simulink model "DetailedHouse"  (R2025a)
settings: Solver=daessc  StartTime=0.0  StopTime=house.operational.datetime.simRunTimeSeconds  MaxStep=60  RelTol=1e-3
PreLoadFcn:
  | run("DetailedHouseParameters.mlx");
undefined symbols (not defined in the file or in its folder): house, value
libraries: fl_lib x36, nesl_utility x14, RoomVolume_lib x12, ExternalWall_lib x5, SolarRadiationAtLocation_lib x1, TemperatureSource_lib x1
CloseFcn:
  | clear house
settings Model: Creator=vikrants  LastModifiedBy=asakhare
settings DataIOCC: ReturnWorkspaceOutputsName=DetailedHouseSimResults

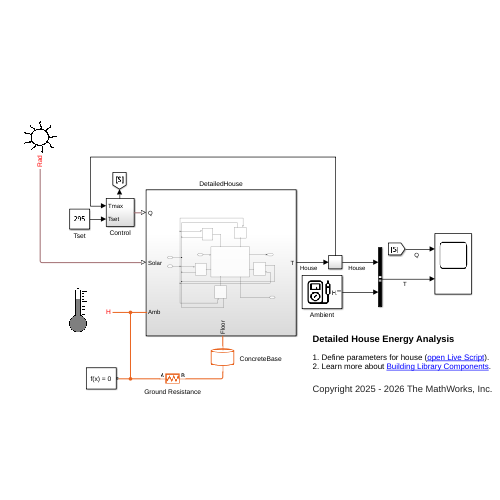
[thumbnail: Simulink's stored preview of the top-level diagram]
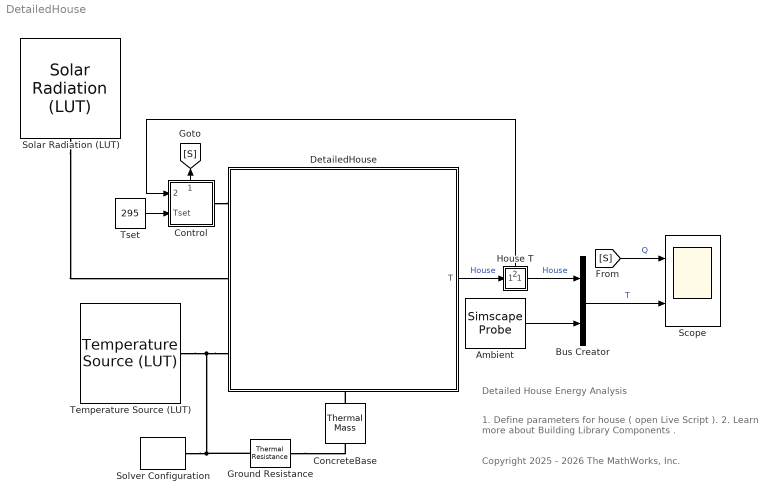
== system DetailedHouse ==
  note: 1. Define parameters for house ( open Live Script ).
      | 2. Learn more about Building Library Components .
  note: Copyright 2025 - 2026 The MathWorks, Inc.
  note: Detailed House Energy Analysis
  Ambient : SimscapeProbe  BoundBlock=326  Variables={H.T}
  Bus Creator : BusCreator  Inputs=2
  ConcreteBase : fl_lib/Thermal/Thermal Elements/Thermal Mass  mass_type=foundation.enum.constant_variable.constant  mass=1000 kg  sp_heat=447 J/(K*kg)  mass_min=1e-6 kg  num_ports=foundation.enum.numPorts2.two  m_specify=off  m_priority=High  m=1 kg  m_nominal_specify=off  m_nominal_value=1  m_nominal_unit=kg  T_specify=on  T_priority=High  T="value(house.heatTransfer.initialT,\"K\") K"  T_nominal_specify=off  T_nominal_value=1  T_nominal_unit=K  Q_specify=off  Q_priority=None  Q=0 W  Q_nominal_specify=off  Q_nominal_value=1  Q_nominal_unit=W
      settings: InternalSimscapePortConfiguration="{\"Bottom\":[],\"Left\":[{\"id\":\"M\",\"label\":\"\",\"type\":\"foundation.thermal.thermal\"}],\"Right\":[{\"id\":\"N\",\"label\":\"\",\"type\":\"foundation.thermal.thermal\"}],\"Top\":[]}"
  Control : Subsystem
      settings: PortSchema="{\"entries\":[{\"content\":{\"sides\":[{\"content\":{\"connectorIds\":[\"LConn1\"]},\"type\":\"ConnectorPlacement.EquallySpacedRectSide\",\"uuid\":\"bf0d3f6c-4199-48ed-9d1b-942d678a196d\"},{\"content\":{\"connectorIds\":[\"In1\",\"In2\"],\"side\":\"RIGHT\"},\"type\":\"ConnectorPlacement.EquallySpacedRectSide\",\"uuid\":\"048b5b2b-ccfc-4083-80b1-51c1896923e2\"},{\"content\":{\"side\":\"TOP\"},\"type\":\"ConnectorPlacement.EquallySpacedRectSide\",\"uuid\":\"550f74ea-2758-4466-8134-2f10276d8ab6\"},{\"content\":{\"connectorIds\":[\"Out1\"],\"side\":\"BOTTOM\"},\"type\":\"ConnectorPlacement.EquallySpacedRectSide\",\"uuid\":\"b8e21315-4710-4fb3-a2ab-c08e79356caa\"}]},\"type\":\"ConnectorPlacement.EquallySpacedConnector\",\"uuid\":\"91aadc23-894a-4dd0-ab72-650090e5f490\"}],\"packageUris\":[\"http://schema.mathworks.com/mf0/Connector/R2020b\"],\"version\":\"1.0\"}"
  DetailedHouse : Subsystem
      settings: PortSchema="{\"entries\":[{\"content\":{\"sides\":[{\"content\":{\"connectorIds\":[\"LConn1\",\"LConn2\",\"LConn3\"]},\"type\":\"ConnectorPlacement.EquallySpacedRectSide\",\"uuid\":\"299cb99e-37c4-4363-a148-c4e2a80bfd54\"},{\"content\":{\"connectorIds\":[\"Out1\"],\"side\":\"RIGHT\"},\"type\":\"ConnectorPlacement.EquallySpacedRectSide\",\"uuid\":\"2fcdd946-1002-4526-8c08-99e8dc6f4c47\"},{\"content\":{\"side\":\"TOP\"},\"type\":\"ConnectorPlacement.EquallySpacedRectSide\",\"uuid\":\"2d615648-e660-4e83-8c42-1b0b4f8091a8\"},{\"content\":{\"connectorIds\":[\"RConn1\"],\"side\":\"BOTTOM\"},\"type\":\"ConnectorPlacement.EquallySpacedRectSide\",\"uuid\":\"84e055a1-92e7-4959-a6d0-9bd398da1db3\"}]},\"type\":\"ConnectorPlacement.EquallySpacedConnector\",\"uuid\":\"3ed9db10-44da-4b23-b671-8dba5af5dcc9\"}],\"packageUris\":[\"http://schema.mathworks.com/mf0/Connector/R2020b\"],\"version\":\"1.0\"}"
  Ground Resistance : fl_lib/Thermal/Thermal Elements/Thermal Resistance  resistance=100 K/W  T_specify=off  T_priority=None  T=0 K  T_nominal_specify=off  T_nominal_value=1  T_nominal_unit=K  Q_specify=off  Q_priority=None  Q=0 W  Q_nominal_specify=off  Q_nominal_value=1  Q_nominal_unit=W
  House T : Subsystem
      settings: PortSchema="{\"entries\":[{\"content\":{\"sides\":[{\"content\":{\"connectorIds\":[\"In1\"]},\"type\":\"ConnectorPlacement.EquallySpacedRectSide\",\"uuid\":\"77a9471e-f475-4272-a324-d9a4c745a553\"},{\"content\":{\"connectorIds\":[\"Out1\"],\"side\":\"RIGHT\"},\"type\":\"ConnectorPlacement.EquallySpacedRectSide\",\"uuid\":\"144991d0-730c-43fd-a2ae-35995e9102ff\"},{\"content\":{\"connectorIds\":[\"Out2\"],\"side\":\"TOP\"},\"type\":\"ConnectorPlacement.EquallySpacedRectSide\",\"uuid\":\"5bc365e2-0ae2-46a9-8284-20be403f9731\"}]},\"type\":\"ConnectorPlacement.EquallySpacedConnector\",\"uuid\":\"845681d4-4f1f-48ee-9a7c-95a2152e9ae6\"}],\"packageUris\":[\"http://schema.mathworks.com/mf0/Connector/R2020b\"],\"version\":\"1.0\"}"
  Scope : Scope  NumInputPorts=2
      settings: ActiveDisplayYMinimum=-520.83333333333337  ActiveDisplayYMaximum=520.83333333333337  YLabel=Q  DataLoggingVariableName=DetailedHouseScopeData
  Solar Radiation (LUT) : SolarRadiationAtLocation_lib/Solar Radiation (LUT)  latitude=house.operational.location.latitude  longitude=house.operational.location.longitude  localTime=house.operational.location.localTime  dayLightS=house.operational.location.daylight  startYear=house.operational.datetime.year  startMonth=house.operational.datetime.month  startDay=house.operational.datetime.day  startHr=house.operational.datetime.hour  numHrsData=house.operational.datetime.numOfHourData  cloudData=cloudCoverLibOption.none  cloudCoverVal=ones(1,ceil(721/24))  interp_method=simscape.enum.interpolation.linear  extrap_method=simscape.enum.extrapolation.nearest
      settings: SourceProductName=Simscape Building Energy Management System Library  InternalSimscapePortConfiguration="{\"Bottom\":[],\"Left\":[],\"Right\":[{\"id\":\"S\",\"label\":\"Rad\",\"type\":\"output\"}],\"Top\":[]}"
  Solver Configuration : nesl_utility/Solver Configuration  PhysicalDomain=network_engine_domain  SubClassName=solver  LeftPortType=input  RightPortType=generic  Tones=[]  Harmonics=[]  SimulateNoise=off  Profile=off  UseLocalSampling=off  EnableSwitchedLinearOptims=on  FrequencyDomain=off  UseCCode=off  RelTol=0.001  AbsTol=0.001  MinStep=1e-09  ToWorkspace=off  RevertToSquareIcSolve=off  NumHomotopyIterations=100  PhasorMode=off  PhasorModeNumHarmonics=1  ConsistencySolver=NEWTON_XTOL_AFTER_FTOL  IndexReductionMethod=DerivativeReplacement  DoDC=off  ResidualTolerance=1e-09  ConsistencyTolSource=GLOBAL  ConsistencyAbsTol=0.001  ConsistencyRelTol=0.001  ConsistencyTolFactor=0.001  UseLocalSolver=off  LocalSolverChoice=NE_BACKWARD_EULER_ADVANCER  ResolveIndetEquations=on  FunctionEvalNumThread=1  LocalSolverSampleTime=0.001  DoFixedCost=off  MaxNonlinIter=3  MaxModeIter=2  ComputeImpulses=off  ImpulseIterations=2  LinearAlgebra=auto  LinearAlgebraNumThread=0  EquationFormulation=NE_TIME_EF  DelaysMemoryBudget=1024  AutomaticFiltering=on  FilteringTimeConstant=0.001  PartitionStorageMethod=AS_NEEDED  PartitionMemoryBudget=1024  PartitionMethod=ROBUST  MultibodyUseLocalSolver=off  MultibodyLocalSolverChoice=ODE1  MultibodyLocalSolverSampleTime=0.001
  Temperature Source (LUT) : TemperatureSource_lib/Temperature Source (LUT)  latitude=house.operational.location.latitude  longitude=house.operational.location.longitude  localTime=house.operational.location.localTime  dayLightS=house.operational.location.daylight  startYear=house.operational.datetime.year  startMonth=house.operational.datetime.month  startDay=house.operational.datetime.day  startHr=house.operational.datetime.hour  numDaysData=house.operational.datetime.numOfDaysData  interp_method=simscape.enum.interpolation.linear  extrap_method=simscape.enum.extrapolation.error  avgDayTvec="value(house.heatTransfer.avgDayTvec,\"K\") K"  pcDayTvar=house.heatTransfer.avgDayTvar  avgNightTvec="value(house.heatTransfer.avgNightTvec,\"K\") K"  pcNightTvar=house.heatTransfer.avgNightTvar
      settings: InternalSimscapePortConfiguration="{\"Bottom\":[],\"Left\":[],\"Right\":[{\"id\":\"H\",\"label\":\"H\",\"type\":\"foundation.thermal.thermal\"}],\"Top\":[]}"
  Tset : Constant  Value=295
  wires:
  DetailedHouse/1(T) -> House T/1(" ")  "House"
  House T/2("    ") -> Control/2(Tmax)
  Tset/1 -> Control/1(Tset)
  Control/1(" ") -> [S]
  Bus Creator/1 -> Scope/2  "T"
  House T/1("  ") -> Bus Creator/1  "House"
  [S] -> Scope/1  "Q"
  Ambient/1 -> Bus Creator/2
  connections:
  Solar Radiation (LUT)/RConn1 -- DetailedHouse/LConn2
  DetailedHouse/LConn3 -- Solver Configuration/RConn1 -- Ground Resistance/LConn1 -- Temperature Source (LUT)/RConn1
  ConcreteBase/LConn1 -- DetailedHouse/RConn1
  Ground Resistance/RConn1 -- ConcreteBase/RConn1
  Control/LConn1 -- DetailedHouse/LConn1

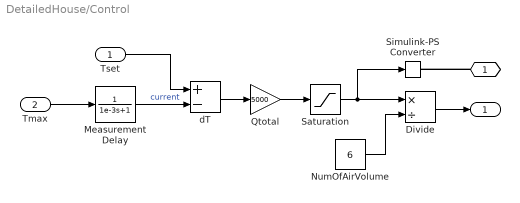
== system DetailedHouse/Control ==
  Tset : Inport
  Tmax : Inport  Port=2
  Divide : Product  Inputs=*/
  Measurement Delay : TransferFcn  Denominator=[1e-3 1]
  NumOfAirVolume : Constant  Value=6
  Qtotal : Gain  Gain=5000
  Saturation : Saturate  UpperLimit=2500  LowerLimit=-2500
  Simulink-PS Converter : nesl_utility/Simulink-PS Converter  PhysicalDomain=network_engine_domain  SubClassName=ps_input  LeftPortType=input  RightPortType=output  PseudoPeriodic=off  Frequencies=[]  NoiseDistribution=none  NoiseParameters=[]  Unit=J/s  AffineConversion=off  FilteringAndDerivatives=provide  SimscapeFilterOrder=1  InputFilterTimeConstant=0.001  UdotUserProvided=0
  dT : Sum  Inputs=+-
  "  " : PMIOPort  Side=Left
  " " : Outport
  wires:
  Tset/1 -> dT/1
  dT/1 -> Qtotal/1
  Qtotal/1 -> Saturation/1
  Saturation/1 -> Divide/1, Simulink-PS Converter/1
  Tmax/1 -> Measurement Delay/1
  Measurement Delay/1 -> dT/2  "current"
  Divide/1 -> " "/1
  NumOfAirVolume/1 -> Divide/2
  connections:
  "  "/RConn1 -- Simulink-PS Converter/RConn1

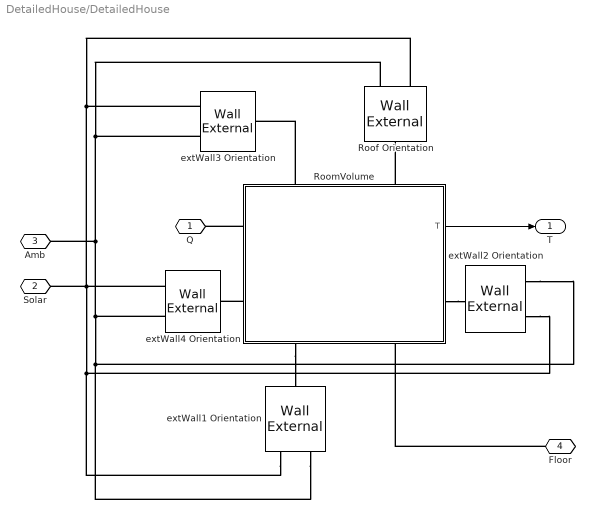
== system DetailedHouse/DetailedHouse ==
  Roof Orientation : ExternalWall_lib/Wall External  extWallModel=wallExternalModelOption.wallSolar  wallLength="value(house.lengthX,\"m\"); m"  wallHeight="value(house.lengthY,\"m\"); m"  wallThickness="house.wall.properties(\"Thickness [m]\",\"Roof\").Variables m"  wallMaterialDen="house.wall.properties(\"Density [kg/m^3]\",\"Roof\").Variables kg/m^3"  wallMaterialCp="house.wall.properties(\"Heat Capacity [J/kg-K]\",\"Roof\").Variables J/(K*kg)"  wallAbsorptivity="house.wall.properties(\"Absorptivity [-]\",\"Roof\").Variables"  wallThermalK="house.wall.properties(\"Thermal Conductivity [W/K-m]\",\"Roof\").Variables W/(K*m)"  winLength=1 m  winHeight=0.5 m  winThickness=0.007 m  winMaterialDen=2500 kg/m^3  winMaterialCp=787 J/(K*kg)  winAbsorptivity=0.35  winThermalK=1 W/(K*m)  winTransmissivity=0.45  ventLength=0.1 m  ventHeight=0.1 m  extToWallHTC="value(house.heatTransfer.externalHTC,\"W/(K*m^2)\") W/(K*m^2)"  intToRoomHTC="value(house.heatTransfer.htc,\"W/(K*m^2)\") W/(K*m^2)"  iniT="value(house.heatTransfer.initialT,\"K\") K"  latitude=house.operational.location.latitude  longitude=house.operational.location.longitude  localTime=house.operational.location.localTime  dayLightS=house.operational.location.daylight  surfAngle=0 deg  surfUnitV=[0, -1]  startYear=house.operational.datetime.year  startMonth=house.operational.datetime.month  startDay=house.operational.datetime.day  startHr=house.operational.datetime.hour  numHrsData=house.operational.datetime.numOfHourData  interp_method=simscape.enum.interpolation.linear  extrap_method=simscape.enum.extrapolation.error
      settings: InternalSimscapePortConfiguration="{\"Bottom\":[],\"Left\":[{\"id\":\"R\",\"label\":\"Rad\",\"type\":\"input\"},{\"id\":\"A\",\"label\":\"A\",\"type\":\"foundation.thermal.thermal\"}],\"Right\":[{\"id\":\"B\",\"label\":\"B\",\"type\":\"foundation.thermal.thermal\"}],\"Top\":[]}"
  RoomVolume : Subsystem
      settings: PortSchema="{\"entries\":[{\"content\":{\"sides\":[{\"content\":{\"connectorIds\":[\"LConn1\",\"LConn2\"]},\"type\":\"ConnectorPlacement.EquallySpacedRectSide\",\"uuid\":\"bb55eb80-d4a7-43ce-a7a0-972e6a4ef911\"},{\"content\":{\"connectorIds\":[\"Out1\",\"RConn1\"],\"side\":\"RIGHT\"},\"type\":\"ConnectorPlacement.EquallySpacedRectSide\",\"uuid\":\"29951cfd-9715-464b-88ca-0c0ac5d49cc2\"},{\"content\":{\"connectorIds\":[\"LConn3\",\"LConn4\"],\"side\":\"TOP\"},\"type\":\"ConnectorPlacement.EquallySpacedRectSide\",\"uuid\":\"a06c10be-0f38-432f-83ff-ea95edd1594a\"},{\"content\":{\"connectorIds\":[\"RConn2\",\"RConn3\"],\"side\":\"BOTTOM\"},\"type\":\"ConnectorPlacement.EquallySpacedRectSide\",\"uuid\":\"c57a9caa-6d36-48ec-a075-3784b3a7d3f9\"}]},\"type\":\"ConnectorPlacement.EquallySpacedConnector\",\"uuid\":\"940ec8b0-d9b9-4e36-b0c1-d94fb2f52aba\"}],\"packageUris\":[\"http://schema.mathworks.com/mf0/Connector/R2020b\"],\"version\":\"1.0\"}"
  extWall1 Orientation : ExternalWall_lib/Wall External  extWallModel=wallExternalModelOption.wallSolarWinVent  wallLength="value(house.lengthX,\"m\") m"  wallHeight="value(house.lengthZ,\"m\") m"  wallThickness="house.wall.properties(\"Thickness [m]\",\"ExternalWall\").Variables m"  wallMaterialDen="house.wall.properties(\"Density [kg/m^3]\",\"ExternalWall\").Variables kg/m^3"  wallMaterialCp="house.wall.properties(\"Heat Capacity [J/kg-K]\",\"ExternalWall\").Variables J/(K*kg)"  wallAbsorptivity="house.wall.properties(\"Absorptivity [-]\",\"ExternalWall\").Variables"  wallThermalK="house.wall.properties(\"Thermal Conductivity [W/K-m]\",\"ExternalWall\").Variables W/(K*m)"  winLength="sqrt(house.wall.opening.window)*value(house.lengthX,\"m\") m"  winHeight="sqrt(house.wall.opening.window)*value(house.lengthZ,\"m\") m"  winThickness="house.wall.properties(\"Thickness [m]\",\"Window\").Variables m"  winMaterialDen="house.wall.properties(\"Density [kg/m^3]\",\"Window\").Variables kg/m^3"  winMaterialCp="house.wall.properties(\"Heat Capacity [J/kg-K]\",\"Window\").Variables J/(K*kg)"  winAbsorptivity="house.wall.properties(\"Absorptivity [-]\",\"Window\").Variables"  winThermalK="house.wall.properties(\"Thermal Conductivity [W/K-m]\",\"Window\").Variables W/(K*m)"  winTransmissivity="house.wall.properties(\"Transmissivity [-]\",\"Window\").Variables"  ventLength="sqrt(house.wall.opening.vent)*value(house.lengthX,\"m\") m"  ventHeight="sqrt(house.wall.opening.vent)*value(house.lengthZ,\"m\") m"  extToWallHTC="value(house.heatTransfer.externalHTC,\"W/(K*m^2)\") W/(K*m^2)"  intToRoomHTC="value(house.heatTransfer.htc,\"W/(K*m^2)\") W/(K*m^2)"  iniT="value(house.heatTransfer.initialT,\"K\") K"  latitude=house.operational.location.latitude  longitude=house.operational.location.longitude  localTime=house.operational.location.localTime  dayLightS=house.operational.location.daylight  surfAngle=90 deg  surfUnitV=[0, -1]  startYear=house.operational.datetime.year  startMonth=house.operational.datetime.month  startDay=house.operational.datetime.day  startHr=house.operational.datetime.hour  numHrsData=house.operational.datetime.numOfHourData  interp_method=simscape.enum.interpolation.linear  extrap_method=simscape.enum.extrapolation.error
      settings: InternalSimscapePortConfiguration="{\"Bottom\":[],\"Left\":[{\"id\":\"R\",\"label\":\"Rad\",\"type\":\"input\"},{\"id\":\"A\",\"label\":\"A\",\"type\":\"foundation.thermal.thermal\"}],\"Right\":[{\"id\":\"B\",\"label\":\"B\",\"type\":\"foundation.thermal.thermal\"}],\"Top\":[]}"
  extWall2 Orientation : ExternalWall_lib/Wall External  extWallModel=wallExternalModelOption.wallSolarVent  wallLength="value(house.lengthY,\"m\"); m"  wallHeight="value(house.lengthZ,\"m\"); m"  wallThickness="house.wall.properties(\"Thickness [m]\",\"ExternalWall\").Variables m"  wallMaterialDen="house.wall.properties(\"Density [kg/m^3]\",\"ExternalWall\").Variables kg/m^3"  wallMaterialCp="house.wall.properties(\"Heat Capacity [J/kg-K]\",\"ExternalWall\").Variables J/(K*kg)"  wallAbsorptivity="house.wall.properties(\"Absorptivity [-]\",\"ExternalWall\").Variables"  wallThermalK="house.wall.properties(\"Thermal Conductivity [W/K-m]\",\"ExternalWall\").Variables W/(K*m)"  winLength=1 m  winHeight=0.5 m  winThickness=0.007 m  winMaterialDen=2500 kg/m^3  winMaterialCp=787 J/(K*kg)  winAbsorptivity=0.35  winThermalK=1 W/(K*m)  winTransmissivity=0.45  ventLength="sqrt(house.wall.opening.vent)*value(house.lengthY,\"m\") m"  ventHeight="sqrt(house.wall.opening.vent)*value(house.lengthZ,\"m\") m"  extToWallHTC="value(house.heatTransfer.externalHTC,\"W/(K*m^2)\") W/(K*m^2)"  intToRoomHTC="value(house.heatTransfer.htc,\"W/(K*m^2)\") W/(K*m^2)"  iniT="value(house.heatTransfer.initialT,\"K\") K"  latitude=house.operational.location.latitude  longitude=house.operational.location.longitude  localTime=house.operational.location.localTime  dayLightS=house.operational.location.daylight  surfAngle=90 deg  surfUnitV=[1,0]  startYear=house.operational.datetime.year  startMonth=house.operational.datetime.month  startDay=house.operational.datetime.day  startHr=house.operational.datetime.hour  numHrsData=house.operational.datetime.numOfHourData  interp_method=simscape.enum.interpolation.linear  extrap_method=simscape.enum.extrapolation.error
      settings: InternalSimscapePortConfiguration="{\"Bottom\":[],\"Left\":[{\"id\":\"R\",\"label\":\"Rad\",\"type\":\"input\"},{\"id\":\"A\",\"label\":\"A\",\"type\":\"foundation.thermal.thermal\"}],\"Right\":[{\"id\":\"B\",\"label\":\"B\",\"type\":\"foundation.thermal.thermal\"}],\"Top\":[]}"
  extWall3 Orientation : ExternalWall_lib/Wall External  extWallModel=wallExternalModelOption.wallSolar  wallLength="value(house.lengthX,\"m\"); m"  wallHeight="value(house.lengthZ,\"m\"); m"  wallThickness="house.wall.properties(\"Thickness [m]\",\"ExternalWall\").Variables m"  wallMaterialDen="house.wall.properties(\"Density [kg/m^3]\",\"ExternalWall\").Variables kg/m^3"  wallMaterialCp="house.wall.properties(\"Heat Capacity [J/kg-K]\",\"ExternalWall\").Variables J/(K*kg)"  wallAbsorptivity="house.wall.properties(\"Absorptivity [-]\",\"ExternalWall\").Variables"  wallThermalK="house.wall.properties(\"Thermal Conductivity [W/K-m]\",\"ExternalWall\").Variables W/(K*m)"  winLength=1 m  winHeight=0.5 m  winThickness=0.007 m  winMaterialDen=2500 kg/m^3  winMaterialCp=787 J/(K*kg)  winAbsorptivity=0.35  winThermalK=1 W/(K*m)  winTransmissivity=0.45  ventLength=0.1 m  ventHeight=0.1 m  extToWallHTC="value(house.heatTransfer.externalHTC,\"W/(K*m^2)\") W/(K*m^2)"  intToRoomHTC="value(house.heatTransfer.htc,\"W/(K*m^2)\") W/(K*m^2)"  iniT="value(house.heatTransfer.initialT,\"K\") K"  latitude=house.operational.location.latitude  longitude=house.operational.location.longitude  localTime=house.operational.location.localTime  dayLightS=house.operational.location.daylight  surfAngle=90 deg  surfUnitV=[0, 1]  startYear=house.operational.datetime.year  startMonth=house.operational.datetime.month  startDay=house.operational.datetime.day  startHr=house.operational.datetime.hour  numHrsData=house.operational.datetime.numOfHourData  interp_method=simscape.enum.interpolation.linear  extrap_method=simscape.enum.extrapolation.error
      settings: InternalSimscapePortConfiguration="{\"Bottom\":[],\"Left\":[{\"id\":\"R\",\"label\":\"Rad\",\"type\":\"input\"},{\"id\":\"A\",\"label\":\"A\",\"type\":\"foundation.thermal.thermal\"}],\"Right\":[{\"id\":\"B\",\"label\":\"B\",\"type\":\"foundation.thermal.thermal\"}],\"Top\":[]}"
  extWall4 Orientation : ExternalWall_lib/Wall External  extWallModel=wallExternalModelOption.wallSolarWin  wallLength="value(house.lengthY,\"m\"); m"  wallHeight="value(house.lengthZ,\"m\"); m"  wallThickness="house.wall.properties(\"Thickness [m]\",\"ExternalWall\").Variables m"  wallMaterialDen="house.wall.properties(\"Density [kg/m^3]\",\"ExternalWall\").Variables kg/m^3"  wallMaterialCp="house.wall.properties(\"Heat Capacity [J/kg-K]\",\"ExternalWall\").Variables J/(K*kg)"  wallAbsorptivity="house.wall.properties(\"Absorptivity [-]\",\"ExternalWall\").Variables"  wallThermalK="house.wall.properties(\"Thermal Conductivity [W/K-m]\",\"ExternalWall\").Variables W/(K*m)"  winLength="sqrt(house.wall.opening.window)*value(house.lengthY,\"m\") m"  winHeight="sqrt(house.wall.opening.window)*value(house.lengthZ,\"m\") m"  winThickness="house.wall.properties(\"Thickness [m]\",\"Window\").Variables m"  winMaterialDen="house.wall.properties(\"Density [kg/m^3]\",\"Window\").Variables kg/m^3"  winMaterialCp="house.wall.properties(\"Heat Capacity [J/kg-K]\",\"Window\").Variables J/(K*kg)"  winAbsorptivity="house.wall.properties(\"Absorptivity [-]\",\"Window\").Variables"  winThermalK="house.wall.properties(\"Thermal Conductivity [W/K-m]\",\"Window\").Variables W/(K*m)"  winTransmissivity="house.wall.properties(\"Transmissivity [-]\",\"Window\").Variables"  ventLength=0.1 m  ventHeight=0.1 m  extToWallHTC="value(house.heatTransfer.externalHTC,\"W/(K*m^2)\") W/(K*m^2)"  intToRoomHTC="value(house.heatTransfer.htc,\"W/(K*m^2)\") W/(K*m^2)"  iniT="value(house.heatTransfer.initialT,\"K\") K"  latitude=house.operational.location.latitude  longitude=house.operational.location.longitude  localTime=house.operational.location.localTime  dayLightS=house.operational.location.daylight  surfAngle=90 deg  surfUnitV=[-1,0]  startYear=house.operational.datetime.year  startMonth=house.operational.datetime.month  startDay=house.operational.datetime.day  startHr=house.operational.datetime.hour  numHrsData=house.operational.datetime.numOfHourData  interp_method=simscape.enum.interpolation.linear  extrap_method=simscape.enum.extrapolation.error
      settings: InternalSimscapePortConfiguration="{\"Bottom\":[],\"Left\":[{\"id\":\"R\",\"label\":\"Rad\",\"type\":\"input\"},{\"id\":\"A\",\"label\":\"A\",\"type\":\"foundation.thermal.thermal\"}],\"Right\":[{\"id\":\"B\",\"label\":\"B\",\"type\":\"foundation.thermal.thermal\"}],\"Top\":[]}"
  Q : PMIOPort  Side=Left
  Solar : PMIOPort  Port=2  Side=Left
  Amb : PMIOPort  Port=3  Side=Left
  Floor : PMIOPort  Port=4  Side=Right
  T : Outport
  wires:
  RoomVolume/1(T) -> T/1
  connections:
  RoomVolume/LConn1 -- Q/RConn1
  Roof Orientation/LConn2 -- extWall2 Orientation/LConn2 -- extWall1 Orientation/LConn2 -- extWall4 Orientation/LConn2 -- Amb/RConn1 -- extWall3 Orientation/LConn2
  RoomVolume/LConn4 -- Roof Orientation/RConn1
  Solar/RConn1 -- extWall3 Orientation/LConn1 -- Roof Orientation/LConn1 -- extWall4 Orientation/LConn1 -- extWall2 Orientation/LConn1 -- extWall1 Orientation/LConn1
  RoomVolume/RConn2 -- extWall1 Orientation/RConn1
  RoomVolume/RConn1 -- extWall2 Orientation/RConn1
  RoomVolume/LConn3 -- extWall3 Orientation/RConn1
  RoomVolume/LConn2 -- extWall4 Orientation/RConn1
  Floor/RConn1 -- RoomVolume/RConn3

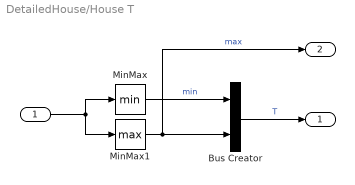
== system DetailedHouse/House T ==
  " " : Inport
  Bus Creator : BusCreator  Inputs=2
  MinMax : MinMax
  MinMax1 : MinMax  Function=max
  "  " : Outport
  "    " : Outport  Port=2
  wires:
  MinMax1/1 -> "    "/1, Bus Creator/2  "max"
  MinMax/1 -> Bus Creator/1  "min"
  " "/1 -> MinMax/1, MinMax1/1
  Bus Creator/1 -> "  "/1  "T"

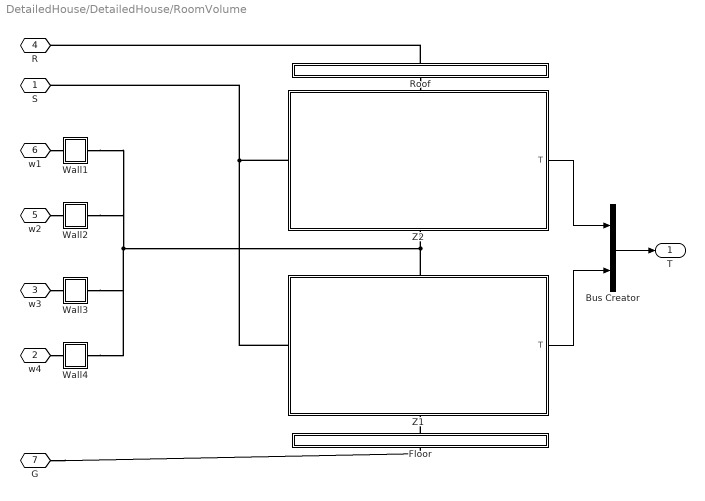
== system DetailedHouse/DetailedHouse/RoomVolume ==
  Bus Creator : BusCreator  Inputs=2
  Floor : Subsystem
  Roof : Subsystem
  Wall1 : Subsystem
  Wall2 : Subsystem
  Wall3 : Subsystem
  Wall4 : Subsystem
  Z1 : Subsystem
      settings: PortSchema="{\"entries\":[{\"content\":{\"sides\":[{\"content\":{\"connectorIds\":[\"LConn1\"]},\"type\":\"ConnectorPlacement.EquallySpacedRectSide\",\"uuid\":\"abda2a5f-a08e-4671-9591-108164548e43\"},{\"content\":{\"connectorIds\":[\"Out1\"],\"side\":\"RIGHT\"},\"type\":\"ConnectorPlacement.EquallySpacedRectSide\",\"uuid\":\"2c40f8a6-94c6-4189-9220-8c37a1cf6112\"},{\"content\":{\"connectorIds\":[\"LConn2\"],\"side\":\"TOP\"},\"type\":\"ConnectorPlacement.EquallySpacedRectSide\",\"uuid\":\"6e9b78ad-d1bd-406b-97de-856c3131d76c\"},{\"content\":{\"connectorIds\":[\"RConn1\"],\"side\":\"BOTTOM\"},\"type\":\"ConnectorPlacement.EquallySpacedRectSide\",\"uuid\":\"1d620671-3a6a-47c3-8dc6-932bf612e3da\"}]},\"type\":\"ConnectorPlacement.EquallySpacedConnector\",\"uuid\":\"389830a2-50d7-49b2-8133-0072793d0210\"}],\"packageUris\":[\"http://schema.mathworks.com/mf0/Connector/R2020b\"],\"version\":\"1.0\"}"
  Z2 : Subsystem
      settings: PortSchema="{\"entries\":[{\"content\":{\"sides\":[{\"content\":{\"connectorIds\":[\"LConn1\"]},\"type\":\"ConnectorPlacement.EquallySpacedRectSide\",\"uuid\":\"abda2a5f-a08e-4671-9591-108164548e43\"},{\"content\":{\"connectorIds\":[\"Out1\"],\"side\":\"RIGHT\"},\"type\":\"ConnectorPlacement.EquallySpacedRectSide\",\"uuid\":\"2c40f8a6-94c6-4189-9220-8c37a1cf6112\"},{\"content\":{\"connectorIds\":[\"LConn2\"],\"side\":\"TOP\"},\"type\":\"ConnectorPlacement.EquallySpacedRectSide\",\"uuid\":\"6e9b78ad-d1bd-406b-97de-856c3131d76c\"},{\"content\":{\"connectorIds\":[\"RConn1\"],\"side\":\"BOTTOM\"},\"type\":\"ConnectorPlacement.EquallySpacedRectSide\",\"uuid\":\"1d620671-3a6a-47c3-8dc6-932bf612e3da\"}]},\"type\":\"ConnectorPlacement.EquallySpacedConnector\",\"uuid\":\"389830a2-50d7-49b2-8133-0072793d0210\"}],\"packageUris\":[\"http://schema.mathworks.com/mf0/Connector/R2020b\"],\"version\":\"1.0\"}"
  S : PMIOPort  Side=Left
  w4 : PMIOPort  Port=2  Side=Left
  w3 : PMIOPort  Port=3  Side=Left
  R : PMIOPort  Port=4  Side=Left
  w2 : PMIOPort  Port=5  Side=Right
  w1 : PMIOPort  Port=6  Side=Right
  G : PMIOPort  Port=7  Side=Right
  T : Outport
  wires:
  Z2/1(T) -> Bus Creator/1
  Z1/1(T) -> Bus Creator/2
  Bus Creator/1 -> T/1
  connections:
  Z1/LConn2 -- Wall2/RConn1 -- Wall1/RConn1 -- Wall4/RConn1 -- Wall3/RConn1 -- Z2/RConn1
  Roof/RConn1 -- Z2/LConn2
  Floor/RConn1 -- Z1/RConn1
  G/RConn1 -- Floor/LConn1
  Z2/LConn1 -- S/RConn1 -- Z1/LConn1
  Roof/LConn1 -- R/RConn1
  w1/RConn1 -- Wall1/LConn1
  w2/RConn1 -- Wall2/LConn1
  w3/RConn1 -- Wall3/LConn1
  w4/RConn1 -- Wall4/LConn1

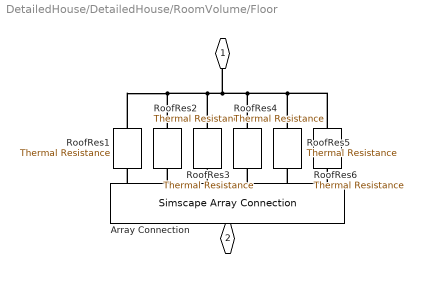
== system DetailedHouse/DetailedHouse/RoomVolume/Floor ==
  Array Connection : SimscapeArrayConnection  Domain=foundation.thermal.thermal  ConcatenateDimension=1  NumScalarElements=6
  RoofRes{1..6} (6 alike) : fl_lib/Thermal/Thermal Elements/Thermal Resistance  resistance=1 K/W  T_specify=off  T_priority=None  T=0 K  T_nominal_specify=off  T_nominal_value=1  T_nominal_unit=K  Q_specify=off  Q_priority=None  Q=0 W  Q_nominal_specify=off  Q_nominal_value=1  Q_nominal_unit=W
  " " : PMIOPort  Side=Left
  "   " : PMIOPort  Port=2  Side=Right
  connections:
  RoofRes1/LConn1 -- RoofRes6/LConn1 -- RoofRes5/LConn1 -- RoofRes4/LConn1 -- " "/RConn1 -- RoofRes3/LConn1 -- RoofRes2/LConn1
  Array Connection/LConn1 -- RoofRes1/RConn1
  Array Connection/LConn2 -- RoofRes2/RConn1
  Array Connection/LConn3 -- RoofRes3/RConn1
  Array Connection/LConn4 -- RoofRes4/RConn1
  Array Connection/LConn5 -- RoofRes5/RConn1
  Array Connection/LConn6 -- RoofRes6/RConn1
  "   "/RConn1 -- Array Connection/RConn1

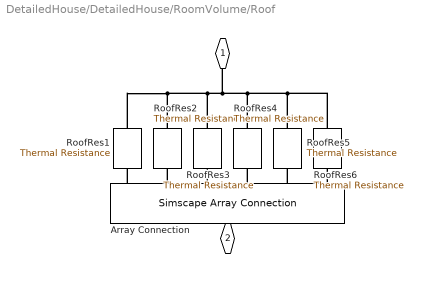
== system DetailedHouse/DetailedHouse/RoomVolume/Roof ==
  Array Connection : SimscapeArrayConnection  Domain=foundation.thermal.thermal  ConcatenateDimension=1  NumScalarElements=6
  RoofRes{1..6} (6 alike) : fl_lib/Thermal/Thermal Elements/Thermal Resistance  resistance=1 K/W  T_specify=off  T_priority=None  T=0 K  T_nominal_specify=off  T_nominal_value=1  T_nominal_unit=K  Q_specify=off  Q_priority=None  Q=0 W  Q_nominal_specify=off  Q_nominal_value=1  Q_nominal_unit=W
  " " : PMIOPort  Side=Left
  "   " : PMIOPort  Port=2  Side=Right
  connections:
  RoofRes1/LConn1 -- RoofRes6/LConn1 -- RoofRes5/LConn1 -- RoofRes4/LConn1 -- " "/RConn1 -- RoofRes3/LConn1 -- RoofRes2/LConn1
  Array Connection/LConn1 -- RoofRes1/RConn1
  Array Connection/LConn2 -- RoofRes2/RConn1
  Array Connection/LConn3 -- RoofRes3/RConn1
  Array Connection/LConn4 -- RoofRes4/RConn1
  Array Connection/LConn5 -- RoofRes5/RConn1
  Array Connection/LConn6 -- RoofRes6/RConn1
  "   "/RConn1 -- Array Connection/RConn1

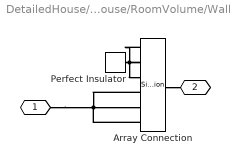
== system DetailedHouse/DetailedHouse/RoomVolume/Wall1 ==
  Array Connection : SimscapeArrayConnection  Domain=foundation.thermal.thermal  ConcatenateDimension=1  NumScalarElements=6
  Perfect Insulator : fl_lib/Thermal/Thermal Elements/Perfect Insulator  T_specify=off  T_priority=None  T=293.15 K  T_nominal_specify=off  T_nominal_value=1  T_nominal_unit=K
  " " : PMIOPort  Side=Left
  "  " : PMIOPort  Port=2  Side=Right
  connections:
  Array Connection/LConn2 -- Array Connection/LConn3 -- Perfect Insulator/LConn1 -- Array Connection/LConn1
  Array Connection/RConn1 -- "  "/RConn1
  " "/RConn1 -- Array Connection/LConn5 -- Array Connection/LConn6 -- Array Connection/LConn4

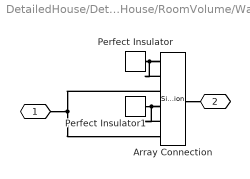
== system DetailedHouse/DetailedHouse/RoomVolume/Wall2 ==
  Array Connection : SimscapeArrayConnection  Domain=foundation.thermal.thermal  ConcatenateDimension=1  NumScalarElements=6
  Perfect Insulator : fl_lib/Thermal/Thermal Elements/Perfect Insulator  T_specify=off  T_priority=None  T=293.15 K  T_nominal_specify=off  T_nominal_value=1  T_nominal_unit=K
  Perfect Insulator1 : fl_lib/Thermal/Thermal Elements/Perfect Insulator  T_specify=off  T_priority=None  T=293.15 K  T_nominal_specify=off  T_nominal_value=1  T_nominal_unit=K
  " " : PMIOPort  Side=Left
  "  " : PMIOPort  Port=2  Side=Right
  connections:
  " "/RConn1 -- Array Connection/LConn6 -- Array Connection/LConn3
  Perfect Insulator/LConn1 -- Array Connection/LConn2 -- Array Connection/LConn1
  Array Connection/RConn1 -- "  "/RConn1
  Perfect Insulator1/LConn1 -- Array Connection/LConn5 -- Array Connection/LConn4

== system DetailedHouse/DetailedHouse/RoomVolume/Wall3 ==
  Array Connection : SimscapeArrayConnection  Domain=foundation.thermal.thermal  ConcatenateDimension=1  NumScalarElements=6
  Perfect Insulator : fl_lib/Thermal/Thermal Elements/Perfect Insulator  T_specify=off  T_priority=None  T=293.15 K  T_nominal_specify=off  T_nominal_value=1  T_nominal_unit=K
  " " : PMIOPort  Side=Left
  "  " : PMIOPort  Port=2  Side=Right
  connections:
  Array Connection/RConn1 -- "  "/RConn1
  Perfect Insulator/LConn1 -- Array Connection/LConn6 -- Array Connection/LConn4 -- Array Connection/LConn5
  " "/RConn1 -- Array Connection/LConn3 -- Array Connection/LConn2 -- Array Connection/LConn1

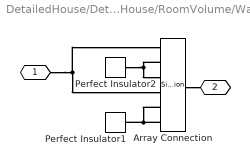
== system DetailedHouse/DetailedHouse/RoomVolume/Wall4 ==
  Array Connection : SimscapeArrayConnection  Domain=foundation.thermal.thermal  ConcatenateDimension=1  NumScalarElements=6
  Perfect Insulator1 : fl_lib/Thermal/Thermal Elements/Perfect Insulator  T_specify=off  T_priority=None  T=293.15 K  T_nominal_specify=off  T_nominal_value=1  T_nominal_unit=K
  Perfect Insulator2 : fl_lib/Thermal/Thermal Elements/Perfect Insulator  T_specify=off  T_priority=None  T=293.15 K  T_nominal_specify=off  T_nominal_value=1  T_nominal_unit=K
  " " : PMIOPort  Side=Left
  "  " : PMIOPort  Port=2  Side=Right
  connections:
  Array Connection/RConn1 -- "  "/RConn1
  Array Connection/LConn5 -- Perfect Insulator1/LConn1 -- Array Connection/LConn6
  " "/RConn1 -- Array Connection/LConn4 -- Array Connection/LConn1
  Perfect Insulator2/LConn1 -- Array Connection/LConn3 -- Array Connection/LConn2

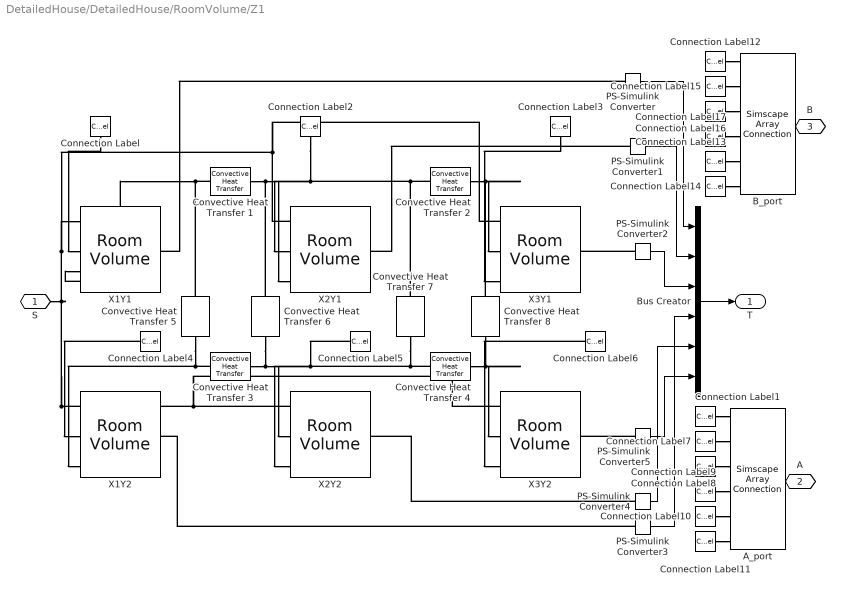
== system DetailedHouse/DetailedHouse/RoomVolume/Z1 ==
  A_port : SimscapeArrayConnection  Domain=foundation.thermal.thermal  ConcatenateDimension=1  NumScalarElements=6
  B_port : SimscapeArrayConnection  Domain=foundation.thermal.thermal  ConcatenateDimension=1  NumScalarElements=6
  Bus Creator : BusCreator  Inputs=6
  Connection Label : ConnectionLabel  Label=A1
  Connection Label1 : ConnectionLabel  Label=A1
  Connection Label10 : ConnectionLabel  Label=A5
  Connection Label11 : ConnectionLabel  Label=A6
  Connection Label12 : ConnectionLabel  Label=A1
  Connection Label13 : ConnectionLabel  Label=A5
  Connection Label14 : ConnectionLabel  Label=A6
  Connection Label15 : ConnectionLabel  Label=A2
  Connection Label16 : ConnectionLabel  Label=A3
  Connection Label17 : ConnectionLabel  Label=A4
  Connection Label2 : ConnectionLabel  Label=A2
  Connection Label3 : ConnectionLabel  Label=A3
  Connection Label4 : ConnectionLabel  Label=A4
  Connection Label5 : ConnectionLabel  Label=A5
  Connection Label6 : ConnectionLabel  Label=A6
  Connection Label7 : ConnectionLabel  Label=A2
  Connection Label8 : ConnectionLabel  Label=A3
  Connection Label9 : ConnectionLabel  Label=A4
  Convective Heat Transfer {1..4} (4 alike) : fl_lib/Thermal/Thermal Elements/Convective Heat Transfer  thermal_type=foundation.enum.constant_variable.constant  area="value(house.lengthY,\"m\")*value(house.lengthZ,\"m\")/(2*2) m^2"  heat_tr_coeff="value(house.heatTransfer.htc,\"W/(K*m^2)\") W/(K*m^2)"  min_heat_tr_coeff=1e-3 W/(K*m^2)  T_specify=off  T_priority=None  T=0 K  T_nominal_specify=off  T_nominal_value=1  T_nominal_unit=K  Q_specify=off  Q_priority=None  Q=0 W  Q_nominal_specify=off  Q_nominal_value=1  Q_nominal_unit=W
  Convective Heat Transfer {5..8} (4 alike) : fl_lib/Thermal/Thermal Elements/Convective Heat Transfer  thermal_type=foundation.enum.constant_variable.constant  area="value(house.lengthX,\"m\")*value(house.lengthZ,\"m\")/(3*2) m^2"  heat_tr_coeff="value(house.heatTransfer.htc,\"W/(K*m^2)\") W/(K*m^2)"  min_heat_tr_coeff=1e-3 W/(K*m^2)  T_specify=off  T_priority=None  T=0 K  T_nominal_specify=off  T_nominal_value=1  T_nominal_unit=K  Q_specify=off  Q_priority=None  Q=0 W  Q_nominal_specify=off  Q_nominal_value=1  Q_nominal_unit=W
  PS-Simulink Converter{,1..5} (6 alike) : nesl_utility/PS-Simulink Converter  PhysicalDomain=network_engine_domain  SubClassName=ps_output  LeftPortType=input  RightPortType=output  PseudoPeriodic=off  Frequencies=[]  VectorFormat=inherit  Unit=inherit  AffineConversion=off
  X1Y1 : RoomVolume_lib/Room Volume  N1=1  N2=1  iniT=300 K  length="value(house.lengthX,\"m\")/3 m"  width="value(house.lengthY,\"m\")/2 m"  height="value(house.lengthZ,\"m\")/2 m"
      settings: InternalSimscapePortConfiguration="{\"Bottom\":[],\"Left\":[{\"id\":\"S\",\"label\":\"S\",\"type\":\"input\"}],\"Right\":[{\"id\":\"T\",\"label\":\"T\",\"type\":\"output\"}],\"Top\":[{\"id\":\"M1\",\"label\":\"M1\",\"type\":\"foundation.thermal.thermal\"},{\"id\":\"M2\",\"label\":\"M2\",\"type\":\"foundation.thermal.thermal\"}]}"
  X1Y2 : RoomVolume_lib/Room Volume  N1=1  N2=1  iniT=300 K  length="value(house.lengthX,\"m\")/3 m"  width="value(house.lengthY,\"m\")/2 m"  height="value(house.lengthZ,\"m\")/2 m"
      settings: InternalSimscapePortConfiguration="{\"Bottom\":[],\"Left\":[{\"id\":\"S\",\"label\":\"S\",\"type\":\"input\"}],\"Right\":[{\"id\":\"T\",\"label\":\"T\",\"type\":\"output\"}],\"Top\":[{\"id\":\"M1\",\"label\":\"M1\",\"type\":\"foundation.thermal.thermal\"},{\"id\":\"M2\",\"label\":\"M2\",\"type\":\"foundation.thermal.thermal\"}]}"
  X2Y1 : RoomVolume_lib/Room Volume  N1=1  N2=1  iniT=300 K  length="value(house.lengthX,\"m\")/3 m"  width="value(house.lengthY,\"m\")/2 m"  height="value(house.lengthZ,\"m\")/2 m"
      settings: InternalSimscapePortConfiguration="{\"Bottom\":[],\"Left\":[{\"id\":\"S\",\"label\":\"S\",\"type\":\"input\"}],\"Right\":[{\"id\":\"T\",\"label\":\"T\",\"type\":\"output\"}],\"Top\":[{\"id\":\"M1\",\"label\":\"M1\",\"type\":\"foundation.thermal.thermal\"},{\"id\":\"M2\",\"label\":\"M2\",\"type\":\"foundation.thermal.thermal\"}]}"
  X2Y2 : RoomVolume_lib/Room Volume  N1=1  N2=1  iniT=300 K  length="value(house.lengthX,\"m\")/3 m"  width="value(house.lengthY,\"m\")/2 m"  height="value(house.lengthZ,\"m\")/2 m"
      settings: InternalSimscapePortConfiguration="{\"Bottom\":[],\"Left\":[{\"id\":\"S\",\"label\":\"S\",\"type\":\"input\"}],\"Right\":[{\"id\":\"T\",\"label\":\"T\",\"type\":\"output\"}],\"Top\":[{\"id\":\"M1\",\"label\":\"M1\",\"type\":\"foundation.thermal.thermal\"},{\"id\":\"M2\",\"label\":\"M2\",\"type\":\"foundation.thermal.thermal\"}]}"
  X3Y1 : RoomVolume_lib/Room Volume  N1=1  N2=1  iniT=300 K  length="value(house.lengthX,\"m\")/3 m"  width="value(house.lengthY,\"m\")/2 m"  height="value(house.lengthZ,\"m\")/2 m"
      settings: InternalSimscapePortConfiguration="{\"Bottom\":[],\"Left\":[{\"id\":\"S\",\"label\":\"S\",\"type\":\"input\"}],\"Right\":[{\"id\":\"T\",\"label\":\"T\",\"type\":\"output\"}],\"Top\":[{\"id\":\"M1\",\"label\":\"M1\",\"type\":\"foundation.thermal.thermal\"},{\"id\":\"M2\",\"label\":\"M2\",\"type\":\"foundation.thermal.thermal\"}]}"
  X3Y2 : RoomVolume_lib/Room Volume  N1=1  N2=1  iniT=300 K  length="value(house.lengthX,\"m\")/3 m"  width="value(house.lengthY,\"m\")/2 m"  height="value(house.lengthZ,\"m\")/2 m"
      settings: InternalSimscapePortConfiguration="{\"Bottom\":[],\"Left\":[{\"id\":\"S\",\"label\":\"S\",\"type\":\"input\"}],\"Right\":[{\"id\":\"T\",\"label\":\"T\",\"type\":\"output\"}],\"Top\":[{\"id\":\"M1\",\"label\":\"M1\",\"type\":\"foundation.thermal.thermal\"},{\"id\":\"M2\",\"label\":\"M2\",\"type\":\"foundation.thermal.thermal\"}]}"
  S : PMIOPort  Side=Left
  A : PMIOPort  Port=2  Side=Left
  B : PMIOPort  Port=3  Side=Right
  T : Outport
  wires:
  PS-Simulink Converter/1 -> Bus Creator/1
  PS-Simulink Converter1/1 -> Bus Creator/2
  PS-Simulink Converter2/1 -> Bus Creator/3
  PS-Simulink Converter3/1 -> Bus Creator/4
  PS-Simulink Converter4/1 -> Bus Creator/5
  PS-Simulink Converter5/1 -> Bus Creator/6
  Bus Creator/1 -> T/1
  connections:
  Convective Heat Transfer 8/RConn1 -- Convective Heat Transfer 4/RConn1 -- X3Y2/LConn2
  Convective Heat Transfer 6/RConn1 -- Convective Heat Transfer 3/RConn1 -- Connection Label5/LConn1 -- X2Y2/LConn2
  Convective Heat Transfer 7/LConn1 -- Convective Heat Transfer 2/LConn1 -- X2Y1/LConn3
  Convective Heat Transfer 5/LConn1 -- X1Y1/LConn3 -- Convective Heat Transfer 1/LConn1
  Convective Heat Transfer 8/LConn1 -- X3Y1/LConn2 -- Convective Heat Transfer 2/RConn1
  PS-Simulink Converter1/LConn1 -- X2Y1/RConn1
  PS-Simulink Converter3/LConn1 -- X1Y2/RConn1
  PS-Simulink Converter5/LConn1 -- X3Y2/RConn1
  PS-Simulink Converter/LConn1 -- X1Y1/RConn1
  Convective Heat Transfer 5/RConn1 -- Convective Heat Transfer 3/LConn1 -- X1Y2/LConn3
  PS-Simulink Converter2/LConn1 -- X3Y1/RConn1
  PS-Simulink Converter4/LConn1 -- X2Y2/RConn1
  S/RConn1 -- X1Y2/LConn1 -- X2Y2/LConn1 -- X3Y2/LConn1 -- X1Y1/LConn1 -- X2Y1/LConn1 -- X3Y1/LConn1
  Connection Label1/LConn1 -- A_port/LConn1
  A/RConn1 -- A_port/RConn1
  Connection Label7/LConn1 -- A_port/LConn2
  Connection Label9/LConn1 -- A_port/LConn4
  Connection Label11/LConn1 -- A_port/LConn6
  Connection Label10/LConn1 -- A_port/LConn5
  Connection Label8/LConn1 -- A_port/LConn3
  B/RConn1 -- B_port/RConn1
  Connection Label14/LConn1 -- B_port/LConn6
  Connection Label12/LConn1 -- B_port/LConn1
  Connection Label16/LConn1 -- B_port/LConn3
  Connection Label13/LConn1 -- B_port/LConn5
  Connection Label17/LConn1 -- B_port/LConn4
  Connection Label15/LConn1 -- B_port/LConn2
  Connection Label/LConn1 -- X1Y1/LConn2
  Convective Heat Transfer 6/LConn1 -- Connection Label2/LConn1 -- X2Y1/LConn2 -- Convective Heat Transfer 1/RConn1
  Connection Label3/LConn1 -- X3Y1/LConn3
  Connection Label4/LConn1 -- X1Y2/LConn2
  Convective Heat Transfer 7/RConn1 -- X2Y2/LConn3 -- Convective Heat Transfer 4/LConn1
  Connection Label6/LConn1 -- X3Y2/LConn3

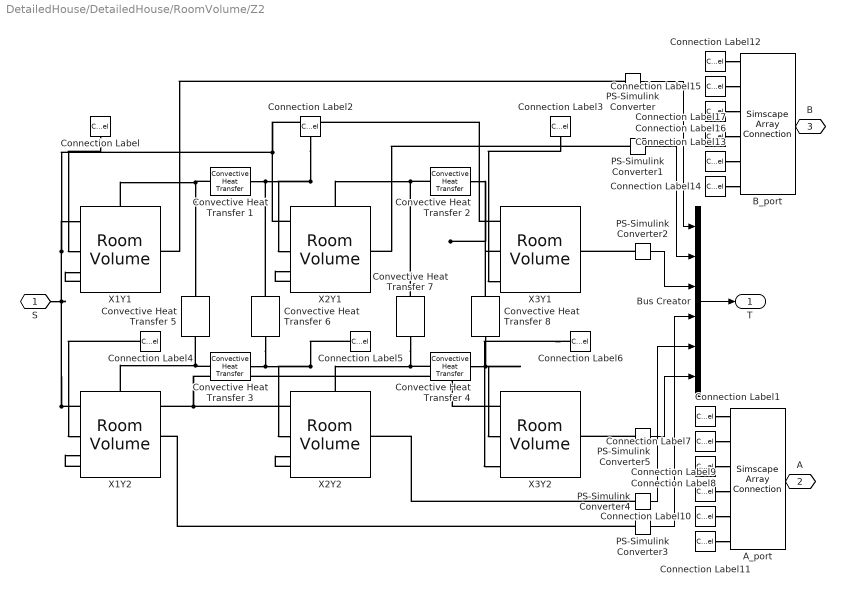
== system DetailedHouse/DetailedHouse/RoomVolume/Z2 ==
  A_port : SimscapeArrayConnection  Domain=foundation.thermal.thermal  ConcatenateDimension=1  NumScalarElements=6
  B_port : SimscapeArrayConnection  Domain=foundation.thermal.thermal  ConcatenateDimension=1  NumScalarElements=6
  Bus Creator : BusCreator  Inputs=6
  Connection Label : ConnectionLabel  Label=A1
  Connection Label1 : ConnectionLabel  Label=A1
  Connection Label10 : ConnectionLabel  Label=A5
  Connection Label11 : ConnectionLabel  Label=A6
  Connection Label12 : ConnectionLabel  Label=A1
  Connection Label13 : ConnectionLabel  Label=A5
  Connection Label14 : ConnectionLabel  Label=A6
  Connection Label15 : ConnectionLabel  Label=A2
  Connection Label16 : ConnectionLabel  Label=A3
  Connection Label17 : ConnectionLabel  Label=A4
  Connection Label2 : ConnectionLabel  Label=A2
  Connection Label3 : ConnectionLabel  Label=A3
  Connection Label4 : ConnectionLabel  Label=A4
  Connection Label5 : ConnectionLabel  Label=A5
  Connection Label6 : ConnectionLabel  Label=A6
  Connection Label7 : ConnectionLabel  Label=A2
  Connection Label8 : ConnectionLabel  Label=A3
  Connection Label9 : ConnectionLabel  Label=A4
  Convective Heat Transfer {1..4} (4 alike) : fl_lib/Thermal/Thermal Elements/Convective Heat Transfer  thermal_type=foundation.enum.constant_variable.constant  area="value(house.lengthY,\"m\")*value(house.lengthZ,\"m\")/(2*2) m^2"  heat_tr_coeff="value(house.heatTransfer.htc,\"W/(K*m^2)\") W/(K*m^2)"  min_heat_tr_coeff=1e-3 W/(K*m^2)  T_specify=off  T_priority=None  T=0 K  T_nominal_specify=off  T_nominal_value=1  T_nominal_unit=K  Q_specify=off  Q_priority=None  Q=0 W  Q_nominal_specify=off  Q_nominal_value=1  Q_nominal_unit=W
  Convective Heat Transfer {5..8} (4 alike) : fl_lib/Thermal/Thermal Elements/Convective Heat Transfer  thermal_type=foundation.enum.constant_variable.constant  area="value(house.lengthX,\"m\")*value(house.lengthZ,\"m\")/(3*2) m^2"  heat_tr_coeff="value(house.heatTransfer.htc,\"W/(K*m^2)\") W/(K*m^2)"  min_heat_tr_coeff=1e-3 W/(K*m^2)  T_specify=off  T_priority=None  T=0 K  T_nominal_specify=off  T_nominal_value=1  T_nominal_unit=K  Q_specify=off  Q_priority=None  Q=0 W  Q_nominal_specify=off  Q_nominal_value=1  Q_nominal_unit=W
  PS-Simulink Converter{,1..5} (6 alike) : nesl_utility/PS-Simulink Converter  PhysicalDomain=network_engine_domain  SubClassName=ps_output  LeftPortType=input  RightPortType=output  PseudoPeriodic=off  Frequencies=[]  VectorFormat=inherit  Unit=inherit  AffineConversion=off
  X1Y1 : RoomVolume_lib/Room Volume  N1=1  N2=1  iniT=300 K  length="value(house.lengthX,\"m\")/3 m"  width="value(house.lengthY,\"m\")/2 m"  height="value(house.lengthZ,\"m\")/2 m"
      settings: InternalSimscapePortConfiguration="{\"Bottom\":[],\"Left\":[{\"id\":\"S\",\"label\":\"S\",\"type\":\"input\"}],\"Right\":[{\"id\":\"T\",\"label\":\"T\",\"type\":\"output\"}],\"Top\":[{\"id\":\"M1\",\"label\":\"M1\",\"type\":\"foundation.thermal.thermal\"},{\"id\":\"M2\",\"label\":\"M2\",\"type\":\"foundation.thermal.thermal\"}]}"
  X1Y2 : RoomVolume_lib/Room Volume  N1=1  N2=1  iniT=300 K  length="value(house.lengthX,\"m\")/3 m"  width="value(house.lengthY,\"m\")/2 m"  height="value(house.lengthZ,\"m\")/2 m"
      settings: InternalSimscapePortConfiguration="{\"Bottom\":[],\"Left\":[{\"id\":\"S\",\"label\":\"S\",\"type\":\"input\"}],\"Right\":[{\"id\":\"T\",\"label\":\"T\",\"type\":\"output\"}],\"Top\":[{\"id\":\"M1\",\"label\":\"M1\",\"type\":\"foundation.thermal.thermal\"},{\"id\":\"M2\",\"label\":\"M2\",\"type\":\"foundation.thermal.thermal\"}]}"
  X2Y1 : RoomVolume_lib/Room Volume  N1=1  N2=1  iniT=300 K  length="value(house.lengthX,\"m\")/3 m"  width="value(house.lengthY,\"m\")/2 m"  height="value(house.lengthZ,\"m\")/2 m"
      settings: InternalSimscapePortConfiguration="{\"Bottom\":[],\"Left\":[{\"id\":\"S\",\"label\":\"S\",\"type\":\"input\"}],\"Right\":[{\"id\":\"T\",\"label\":\"T\",\"type\":\"output\"}],\"Top\":[{\"id\":\"M1\",\"label\":\"M1\",\"type\":\"foundation.thermal.thermal\"},{\"id\":\"M2\",\"label\":\"M2\",\"type\":\"foundation.thermal.thermal\"}]}"
  X2Y2 : RoomVolume_lib/Room Volume  N1=1  N2=1  iniT=300 K  length="value(house.lengthX,\"m\")/3 m"  width="value(house.lengthY,\"m\")/2 m"  height="value(house.lengthZ,\"m\")/2 m"
      settings: InternalSimscapePortConfiguration="{\"Bottom\":[],\"Left\":[{\"id\":\"S\",\"label\":\"S\",\"type\":\"input\"}],\"Right\":[{\"id\":\"T\",\"label\":\"T\",\"type\":\"output\"}],\"Top\":[{\"id\":\"M1\",\"label\":\"M1\",\"type\":\"foundation.thermal.thermal\"},{\"id\":\"M2\",\"label\":\"M2\",\"type\":\"foundation.thermal.thermal\"}]}"
  X3Y1 : RoomVolume_lib/Room Volume  N1=1  N2=1  iniT=300 K  length="value(house.lengthX,\"m\")/3 m"  width="value(house.lengthY,\"m\")/2 m"  height="value(house.lengthZ,\"m\")/2 m"
      settings: InternalSimscapePortConfiguration="{\"Bottom\":[],\"Left\":[{\"id\":\"S\",\"label\":\"S\",\"type\":\"input\"}],\"Right\":[{\"id\":\"T\",\"label\":\"T\",\"type\":\"output\"}],\"Top\":[{\"id\":\"M1\",\"label\":\"M1\",\"type\":\"foundation.thermal.thermal\"},{\"id\":\"M2\",\"label\":\"M2\",\"type\":\"foundation.thermal.thermal\"}]}"
  X3Y2 : RoomVolume_lib/Room Volume  N1=1  N2=1  iniT=300 K  length="value(house.lengthX,\"m\")/3 m"  width="value(house.lengthY,\"m\")/2 m"  height="value(house.lengthZ,\"m\")/2 m"
      settings: InternalSimscapePortConfiguration="{\"Bottom\":[],\"Left\":[{\"id\":\"S\",\"label\":\"S\",\"type\":\"input\"}],\"Right\":[{\"id\":\"T\",\"label\":\"T\",\"type\":\"output\"}],\"Top\":[{\"id\":\"M1\",\"label\":\"M1\",\"type\":\"foundation.thermal.thermal\"},{\"id\":\"M2\",\"label\":\"M2\",\"type\":\"foundation.thermal.thermal\"}]}"
  S : PMIOPort  Side=Left
  A : PMIOPort  Port=2  Side=Left
  B : PMIOPort  Port=3  Side=Right
  T : Outport
  wires:
  PS-Simulink Converter/1 -> Bus Creator/1
  PS-Simulink Converter1/1 -> Bus Creator/2
  PS-Simulink Converter2/1 -> Bus Creator/3
  PS-Simulink Converter3/1 -> Bus Creator/4
  PS-Simulink Converter4/1 -> Bus Creator/5
  PS-Simulink Converter5/1 -> Bus Creator/6
  Bus Creator/1 -> T/1
  connections:
  Convective Heat Transfer 8/RConn1 -- Convective Heat Transfer 4/RConn1 -- X3Y2/LConn2
  Convective Heat Transfer 6/RConn1 -- Convective Heat Transfer 3/RConn1 -- Connection Label5/LConn1 -- X2Y2/LConn2
  Convective Heat Transfer 7/LConn1 -- X2Y1/LConn3 -- Convective Heat Transfer 2/LConn1
  Connection Label/LConn1 -- X1Y1/LConn2
  X3Y1/LConn2 -- Convective Heat Transfer 8/LConn1 -- Convective Heat Transfer 2/RConn1
  PS-Simulink Converter1/LConn1 -- X2Y1/RConn1
  PS-Simulink Converter3/LConn1 -- X1Y2/RConn1
  PS-Simulink Converter5/LConn1 -- X3Y2/RConn1
  PS-Simulink Converter/LConn1 -- X1Y1/RConn1
  Convective Heat Transfer 3/LConn1 -- X1Y2/LConn3 -- Convective Heat Transfer 5/RConn1
  PS-Simulink Converter2/LConn1 -- X3Y1/RConn1
  PS-Simulink Converter4/LConn1 -- X2Y2/RConn1
  S/RConn1 -- X1Y2/LConn1 -- X2Y2/LConn1 -- X3Y2/LConn1 -- X2Y1/LConn1 -- X3Y1/LConn1 -- X1Y1/LConn1
  Connection Label1/LConn1 -- A_port/LConn1
  A/RConn1 -- A_port/RConn1
  Connection Label7/LConn1 -- A_port/LConn2
  Connection Label9/LConn1 -- A_port/LConn4
  Connection Label11/LConn1 -- A_port/LConn6
  Connection Label10/LConn1 -- A_port/LConn5
  Connection Label8/LConn1 -- A_port/LConn3
  B/RConn1 -- B_port/RConn1
  Connection Label14/LConn1 -- B_port/LConn6
  Connection Label12/LConn1 -- B_port/LConn1
  Connection Label16/LConn1 -- B_port/LConn3
  Connection Label13/LConn1 -- B_port/LConn5
  Connection Label17/LConn1 -- B_port/LConn4
  Connection Label15/LConn1 -- B_port/LConn2
  Convective Heat Transfer 1/LConn1 -- X1Y1/LConn3 -- Convective Heat Transfer 5/LConn1
  Connection Label2/LConn1 -- Convective Heat Transfer 6/LConn1 -- Convective Heat Transfer 1/RConn1 -- X2Y1/LConn2
  Connection Label3/LConn1 -- X3Y1/LConn3
  Connection Label4/LConn1 -- X1Y2/LConn2
  Convective Heat Transfer 7/RConn1 -- X2Y2/LConn3 -- Convective Heat Transfer 4/LConn1
  Connection Label6/LConn1 -- X3Y2/LConn3
